simulink model "Conical_Tank_model"  (R2021a)
settings: Solver=VariableStepAuto  StartTime=0.0  StopTime=10000  RelTol=1e-3
settings Model: Creator=SABARNA  LastModifiedBy=SABARNA
settings DataIOCC: ReturnWorkspaceOutputs=off

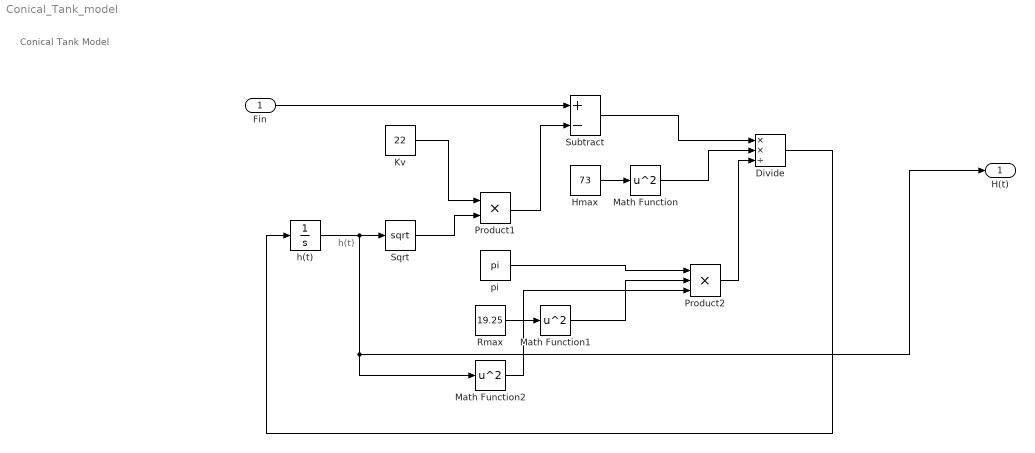
== system Conical_Tank_model ==
  note: h(t)
  note: Conical Tank Model
  Fin : Inport
  Divide : Product  Inputs=**/
  Hmax : Constant  Value=73
  Kv : Constant  Value=22
  Math Function : Math  Operator=square  SaturateOnIntegerOverflow=on
  Math Function1 : Math  Operator=square  SaturateOnIntegerOverflow=on
  Math Function2 : Math  Operator=square  SaturateOnIntegerOverflow=on
  Product1 : Product
  Product2 : Product  Inputs=3
  Rmax : Constant  Value=19.25
  Sqrt : Sqrt  SaturateOnIntegerOverflow=on
  Subtract : Sum  Inputs=+-
  h(t) : Integrator  InitialCondition=10  LimitOutput=on  UpperSaturationLimit=60  LowerSaturationLimit=10
  pi : Constant  Value=pi
  H(t) : Outport
  wires:
  Math Function1/1 -> Product2/2
  Product1/1 -> Subtract/2
  Product2/1 -> Divide/3
  pi/1 -> Product2/1
  Rmax/1 -> Math Function1/1
  Divide/1 -> h(t)/1
  Math Function/1 -> Divide/2
  Subtract/1 -> Divide/1
  Hmax/1 -> Math Function/1
  Sqrt/1 -> Product1/2
  h(t)/1 -> Math Function2/1, H(t)/1, Sqrt/1
  Math Function2/1 -> Product2/3
  Kv/1 -> Product1/1
  Fin/1 -> Subtract/1
